simulink model "untitled1"  (R2019b)
settings: Solver=VariableStepAuto  StartTime=0.0  StopTime=160  RelTol=1e-3
values from neighbouring files (symbols this model uses):
  omega_0 = 0    [apll_attr.m]    (also in apll_const.m; main.m = 700; test.m)
  w_fr = w_r - 700    (= 2)    [main.m]
  w_r = 702    [main.m]
undefined symbols (not defined in the file or in its folder): K_p, K_v
libraries: simulink x2
settings Model: Creator=Elena  LastModifiedBy=Elena

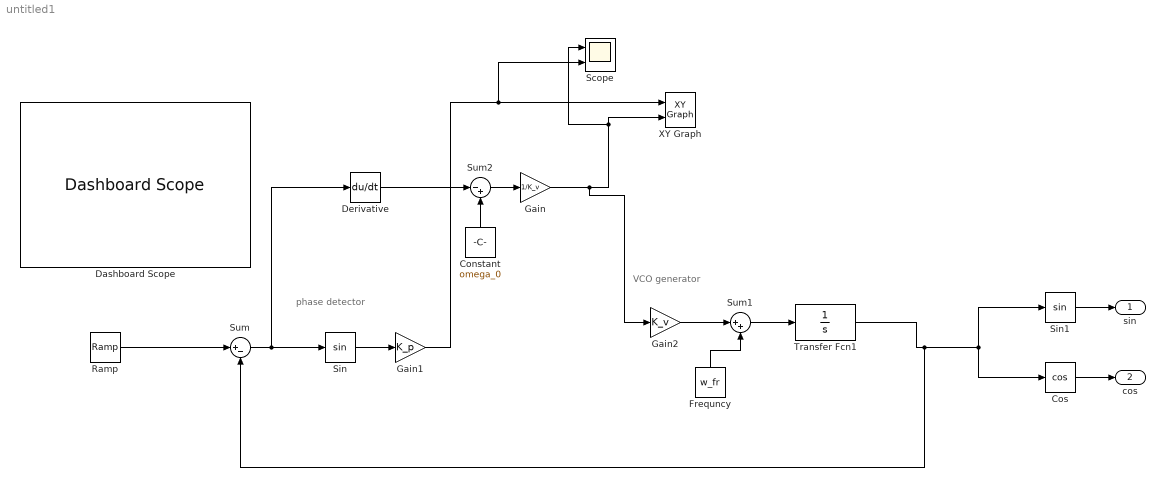
== system untitled1 ==
  note: phase detector
  note: VCO generator
  Constant : Constant  Value=omega_0
  Cos : Trigonometry  Operator=cos
  Dashboard Scope : DashboardScope
  Derivative : Derivative
  Frequncy : Constant  Value=w_fr
  Gain : Gain  Gain=1/K_v
  Gain1 : Gain  Gain=K_p
  Gain2 : Gain  Gain=K_v
  Ramp : simulink/Sources/Ramp  slope=w_r  start=0  InitialOutput=0
  Scope : Scope  NumInputPorts=2
  Sin : Trigonometry
  Sin1 : Trigonometry
  Sum : Sum  Inputs=|+-
  Sum1 : Sum  Inputs=|++
  Sum2 : Sum  Inputs=|-+
  Transfer Fcn1 : TransferFcn  Denominator=[1 0]
  XY Graph : simulink/Sinks/XY Graph  xmin=-1  xmax=1  ymin=1  ymax=1  st=-1
  sin : Outport
  cos : Outport  Port=2
  wires:
  Sum1/1 -> Transfer Fcn1/1
  Sin/1 -> Gain1/1
  Ramp/1 -> Sum/1
  Gain1/1 -> Scope/2, XY Graph/1
  Sin1/1 -> sin/1
  Frequncy/1 -> Sum1/2
  Transfer Fcn1/1 -> Sum/2, Cos/1, Sin1/1
  Cos/1 -> cos/1
  Sum/1 -> Derivative/1, Sin/1
  Constant/1 -> Sum2/2
  Gain/1 -> Gain2/1, Scope/1, XY Graph/2
  Gain2/1 -> Sum1/1
  Sum2/1 -> Gain/1
  Derivative/1 -> Sum2/1
